simulink model "gm_parallel_prediction_and_cost_function_6phase"  (R2022a)
settings: Solver=FixedStepDiscrete  StartTime=0.0  StopTime=10.0  RelTol=1e-3
undefined symbols (not defined in the file or in its folder): f_c, L_d, L_q, L_x, L_y, p, psi_pm, R_ph
libraries: hdlmdlgenlib x2
(part 5 of 8)

== system gm_parallel_prediction_and_cost_function_6phase/Prediction_and_cost_function/Subsystem/Subsystem3 ==
  SampleTime_div_Ld : Inport  OutDataTypeStr=single  PortDimensions=1  SampleTime=1e-08
  SampleTime_div_Lq : Inport  Port=2  OutDataTypeStr=single  PortDimensions=1  SampleTime=1e-08
  SampleTime_div_Lx : Inport  Port=3  OutDataTypeStr=single  PortDimensions=1  SampleTime=1e-08
  SampleTime_div_Ly : Inport  Port=4  OutDataTypeStr=single  PortDimensions=1  SampleTime=1e-08
  d_phase_voltage_per_switching_state : Inport  Port=5  OutDataTypeStr=single  PortDimensions=1  SampleTime=1e-08
  q_phase_voltage_per_switching_state : Inport  Port=6  OutDataTypeStr=single  PortDimensions=1  SampleTime=1e-08
  x_phase_voltage_per_switching_state : Inport  Port=7  OutDataTypeStr=single  PortDimensions=1  SampleTime=1e-08
  y_phase_voltage_per_switching_state : Inport  Port=8  OutDataTypeStr=single  PortDimensions=1  SampleTime=1e-08
  id_k : Inport  Port=9  OutDataTypeStr=single  PortDimensions=1  SampleTime=1e-08
  iq_k : Inport  Port=10  OutDataTypeStr=single  PortDimensions=1  SampleTime=1e-08
  ix_k : Inport  Port=11  OutDataTypeStr=single  PortDimensions=1  SampleTime=1e-08
  iy_k : Inport  Port=12  OutDataTypeStr=single  PortDimensions=1  SampleTime=1e-08
  psiPM : Inport  Port=13  OutDataTypeStr=single  PortDimensions=1  SampleTime=1e-08
  Lq : Inport  Port=14  OutDataTypeStr=single  PortDimensions=1  SampleTime=1e-08
  Ld : Inport  Port=15  OutDataTypeStr=single  PortDimensions=1  SampleTime=1e-08
  Rs : Inport  Port=16  OutDataTypeStr=single  PortDimensions=1  SampleTime=1e-08
  omega_el : Inport  Port=17  OutDataTypeStr=single  PortDimensions=1  SampleTime=1e-08
  Add : Subsystem
      mask Display: disp('NFP\nadd');
  Add1 : Subsystem
      mask Display: disp('NFP\nadd');
  Add2 : Subsystem
      mask Display: disp('NFP\nadd');
  Add3 : Subsystem
      mask Display: disp('NFP\nadd');
  Add4 : Subsystem
      mask Display: disp('NFP\nadd');
  Product1 : Subsystem
      mask Display: disp('NFP\nmul');
  Product10 : Subsystem
      mask Display: disp('NFP\nmul');
  Product11 : Subsystem
      mask Display: disp('NFP\nmul');
  Product2 : Subsystem
      mask Display: disp('NFP\nmul');
  Product3 : Subsystem
      mask Display: disp('NFP\nmul');
  Product31 : Subsystem
      mask Display: disp('NFP\nmul');
  Product4 : Subsystem
      mask Display: disp('NFP\nmul');
  Product5 : Subsystem
      mask Display: disp('NFP\nmul');
  Product6 : Subsystem
      mask Display: disp('NFP\nmul');
  Product7 : Subsystem
      mask Display: disp('NFP\nmul');
  Product8 : Subsystem
      mask Display: disp('NFP\nmul');
  Product9 : Subsystem
      mask Display: disp('NFP\nmul');
  Subtract1_stage2 : Subsystem
      mask Display: disp('NFP\nadd');
  Subtract1_stage3 : Subsystem
      mask Display: disp('NFP\nadd');
  Subtract2 : Subsystem
      mask Display: disp('NFP\nadd');
  Subtract3 : Subsystem
      mask Display: disp('NFP\nadd');
  Subtract_stage2 : Subsystem
      mask Display: disp('NFP\nadd');
  Subtract_stage3 : Subsystem
      mask Display: disp('NFP\nadd');
  delayMatch : Delay  DelayLength=double(18)  InitialCondition=0  SampleTime=1e-08
  delayMatch1 : Delay  DelayLength=double(18)  InitialCondition=0  SampleTime=1e-08
  delayMatch{2,10..11,13,16..31} (20 alike) : Delay  DelayLength=double(6)  InitialCondition=0  SampleTime=1e-08
  delayMatch{5..9,12,14..15} (8 alike) : Delay  DelayLength=double(12)  InitialCondition=0  SampleTime=1e-08
  delayMatch3 : Delay  DelayLength=double(24)  InitialCondition=0  SampleTime=1e-08
  delayMatch4 : Delay  DelayLength=double(24)  InitialCondition=0  SampleTime=1e-08
  id_13 : Outport  SampleTime=1e-08
  iq_13 : Outport  Port=2  SampleTime=1e-08
  ix_13 : Outport  Port=3  SampleTime=1e-08
  iy_13 : Outport  Port=4  SampleTime=1e-08
  wires:
  delayMatch13/1 -> Subtract_stage3/1(In1)
  delayMatch21/1 -> Subtract1_stage3/1(In1)
  delayMatch14/1 -> Product1/1(In1)
  delayMatch22/1 -> Product4/1(In1)
  delayMatch26/1 -> Product8/1(In1)
  delayMatch30/1 -> Product10/1(In1)
  delayMatch11/1 -> Subtract_stage2/1(In1)
  delayMatch17/1 -> Subtract1_stage2/1(In1)
  delayMatch25/1 -> Subtract2/1(In1)
  delayMatch29/1 -> Subtract3/1(In1)
  delayMatch15/1 -> Add/2(In2)
  delayMatch12/1 -> Product31/2(In2)
  delayMatch27/1 -> Add3/2(In2)
  delayMatch31/1 -> Add4/2(In2)
  delayMatch19/1 -> Add2/1(In1)
  delayMatch20/1 -> Product6/1(In1)
  Add/1(Out1) -> id_13/1
  Add1/1(Out1) -> iq_13/1
  Add2/1(Out1) -> Product6/2(In2)
  Add3/1(Out1) -> ix_13/1
  Add4/1(Out1) -> iy_13/1
  Product1/1(Out1) -> Add/1(In1)
  Product10/1(Out1) -> Add4/1(In1)
  Product11/1(Out1) -> Subtract3/2(In2)
  Product2/1(Out1) -> Subtract_stage2/2(In2)
  Product3/1(Out1) -> Product31/1(In1)
  Product31/1(Out1) -> Subtract_stage3/2(In2)
  Product4/1(Out1) -> Add1/1(In1)
  Product5/1(Out1) -> Subtract1_stage2/2(In2)
  Product6/1(Out1) -> Subtract1_stage3/2(In2)
  Product7/1(Out1) -> Add2/2(In2)
  Product8/1(Out1) -> Add3/1(In1)
  Product9/1(Out1) -> Subtract2/2(In2)
  Subtract_stage2/1(Out1) -> delayMatch13/1
  Subtract_stage3/1(Out1) -> Product1/2(In2)
  Subtract1_stage2/1(Out1) -> delayMatch21/1
  Subtract1_stage3/1(Out1) -> Product4/2(In2)
  Subtract2/1(Out1) -> Product8/2(In2)
  Subtract3/1(Out1) -> Product10/2(In2)
  delayMatch23/1 -> Add1/2(In2)
  delayMatch9/1 -> Product3/2(In2)
  delayMatch18/1 -> Product7/2(In2)
  delayMatch10/1 -> Product2/2(In2)
  delayMatch16/1 -> Product5/2(In2)
  delayMatch/1 -> delayMatch14/1
  delayMatch1/1 -> delayMatch15/1
  delayMatch24/1 -> Product9/2(In2)
  delayMatch2/1 -> delayMatch19/1
  delayMatch3/1 -> delayMatch22/1
  delayMatch4/1 -> delayMatch23/1
  delayMatch28/1 -> Product11/2(In2)
  delayMatch5/1 -> delayMatch26/1
  delayMatch6/1 -> delayMatch27/1
  delayMatch7/1 -> delayMatch30/1
  delayMatch8/1 -> delayMatch31/1
  SampleTime_div_Ld/1 -> delayMatch/1
  SampleTime_div_Lq/1 -> delayMatch3/1
  SampleTime_div_Lx/1 -> delayMatch5/1
  SampleTime_div_Ly/1 -> delayMatch7/1
  d_phase_voltage_per_switching_state/1 -> delayMatch11/1
  q_phase_voltage_per_switching_state/1 -> delayMatch17/1
  x_phase_voltage_per_switching_state/1 -> delayMatch25/1
  y_phase_voltage_per_switching_state/1 -> delayMatch29/1
  id_k/1 -> delayMatch1/1, Product7/1(In1), Product2/1(In1)
  iq_k/1 -> delayMatch4/1, Product5/1(In1), delayMatch12/1
  ix_k/1 -> delayMatch6/1, Product9/1(In1)
  iy_k/1 -> delayMatch8/1, Product11/1(In1)
  psiPM/1 -> delayMatch2/1
  Lq/1 -> delayMatch9/1
  Ld/1 -> delayMatch18/1
  Rs/1 -> delayMatch28/1, delayMatch24/1, delayMatch16/1, delayMatch10/1
  omega_el/1 -> Product3/1(In1), delayMatch20/1

== system gm_parallel_prediction_and_cost_function_6phase/Prediction_and_cost_function/Subsystem/Subsystem4 ==
  SampleTime_div_Ld : Inport  OutDataTypeStr=single  PortDimensions=1  SampleTime=1e-08
  SampleTime_div_Lq : Inport  Port=2  OutDataTypeStr=single  PortDimensions=1  SampleTime=1e-08
  SampleTime_div_Lx : Inport  Port=3  OutDataTypeStr=single  PortDimensions=1  SampleTime=1e-08
  SampleTime_div_Ly : Inport  Port=4  OutDataTypeStr=single  PortDimensions=1  SampleTime=1e-08
  d_phase_voltage_per_switching_state : Inport  Port=5  OutDataTypeStr=single  PortDimensions=1  SampleTime=1e-08
  q_phase_voltage_per_switching_state : Inport  Port=6  OutDataTypeStr=single  PortDimensions=1  SampleTime=1e-08
  x_phase_voltage_per_switching_state : Inport  Port=7  OutDataTypeStr=single  PortDimensions=1  SampleTime=1e-08
  y_phase_voltage_per_switching_state : Inport  Port=8  OutDataTypeStr=single  PortDimensions=1  SampleTime=1e-08
  id_k : Inport  Port=9  OutDataTypeStr=single  PortDimensions=1  SampleTime=1e-08
  iq_k : Inport  Port=10  OutDataTypeStr=single  PortDimensions=1  SampleTime=1e-08
  ix_k : Inport  Port=11  OutDataTypeStr=single  PortDimensions=1  SampleTime=1e-08
  iy_k : Inport  Port=12  OutDataTypeStr=single  PortDimensions=1  SampleTime=1e-08
  psiPM : Inport  Port=13  OutDataTypeStr=single  PortDimensions=1  SampleTime=1e-08
  Lq : Inport  Port=14  OutDataTypeStr=single  PortDimensions=1  SampleTime=1e-08
  Ld : Inport  Port=15  OutDataTypeStr=single  PortDimensions=1  SampleTime=1e-08
  Rs : Inport  Port=16  OutDataTypeStr=single  PortDimensions=1  SampleTime=1e-08
  omega_el : Inport  Port=17  OutDataTypeStr=single  PortDimensions=1  SampleTime=1e-08
  Add : Subsystem
      mask Display: disp('NFP\nadd');
  Add1 : Subsystem
      mask Display: disp('NFP\nadd');
  Add2 : Subsystem
      mask Display: disp('NFP\nadd');
  Add3 : Subsystem
      mask Display: disp('NFP\nadd');
  Add4 : Subsystem
      mask Display: disp('NFP\nadd');
  Product1 : Subsystem
      mask Display: disp('NFP\nmul');
  Product10 : Subsystem
      mask Display: disp('NFP\nmul');
  Product11 : Subsystem
      mask Display: disp('NFP\nmul');
  Product2 : Subsystem
      mask Display: disp('NFP\nmul');
  Product3 : Subsystem
      mask Display: disp('NFP\nmul');
  Product31 : Subsystem
      mask Display: disp('NFP\nmul');
  Product4 : Subsystem
      mask Display: disp('NFP\nmul');
  Product5 : Subsystem
      mask Display: disp('NFP\nmul');
  Product6 : Subsystem
      mask Display: disp('NFP\nmul');
  Product7 : Subsystem
      mask Display: disp('NFP\nmul');
  Product8 : Subsystem
      mask Display: disp('NFP\nmul');
  Product9 : Subsystem
      mask Display: disp('NFP\nmul');
  Subtract1_stage2 : Subsystem
      mask Display: disp('NFP\nadd');
  Subtract1_stage3 : Subsystem
      mask Display: disp('NFP\nadd');
  Subtract2 : Subsystem
      mask Display: disp('NFP\nadd');
  Subtract3 : Subsystem
      mask Display: disp('NFP\nadd');
  Subtract_stage2 : Subsystem
      mask Display: disp('NFP\nadd');
  Subtract_stage3 : Subsystem
      mask Display: disp('NFP\nadd');
  delayMatch : Delay  DelayLength=double(18)  InitialCondition=0  SampleTime=1e-08
  delayMatch1 : Delay  DelayLength=double(18)  InitialCondition=0  SampleTime=1e-08
  delayMatch{2,10..11,13,16..31} (20 alike) : Delay  DelayLength=double(6)  InitialCondition=0  SampleTime=1e-08
  delayMatch{5..9,12,14..15} (8 alike) : Delay  DelayLength=double(12)  InitialCondition=0  SampleTime=1e-08
  delayMatch3 : Delay  DelayLength=double(24)  InitialCondition=0  SampleTime=1e-08
  delayMatch4 : Delay  DelayLength=double(24)  InitialCondition=0  SampleTime=1e-08
  id_12 : Outport  SampleTime=1e-08
  iq_12 : Outport  Port=2  SampleTime=1e-08
  ix_12 : Outport  Port=3  SampleTime=1e-08
  iy_12 : Outport  Port=4  SampleTime=1e-08
  wires:
  delayMatch13/1 -> Subtract_stage3/1(In1)
  delayMatch21/1 -> Subtract1_stage3/1(In1)
  delayMatch14/1 -> Product1/1(In1)
  delayMatch22/1 -> Product4/1(In1)
  delayMatch26/1 -> Product8/1(In1)
  delayMatch30/1 -> Product10/1(In1)
  delayMatch11/1 -> Subtract_stage2/1(In1)
  delayMatch17/1 -> Subtract1_stage2/1(In1)
  delayMatch25/1 -> Subtract2/1(In1)
  delayMatch29/1 -> Subtract3/1(In1)
  delayMatch15/1 -> Add/2(In2)
  delayMatch12/1 -> Product31/2(In2)
  delayMatch27/1 -> Add3/2(In2)
  delayMatch31/1 -> Add4/2(In2)
  delayMatch19/1 -> Add2/1(In1)
  delayMatch20/1 -> Product6/1(In1)
  Add/1(Out1) -> id_12/1
  Add1/1(Out1) -> iq_12/1
  Add2/1(Out1) -> Product6/2(In2)
  Add3/1(Out1) -> ix_12/1
  Add4/1(Out1) -> iy_12/1
  Product1/1(Out1) -> Add/1(In1)
  Product10/1(Out1) -> Add4/1(In1)
  Product11/1(Out1) -> Subtract3/2(In2)
  Product2/1(Out1) -> Subtract_stage2/2(In2)
  Product3/1(Out1) -> Product31/1(In1)
  Product31/1(Out1) -> Subtract_stage3/2(In2)
  Product4/1(Out1) -> Add1/1(In1)
  Product5/1(Out1) -> Subtract1_stage2/2(In2)
  Product6/1(Out1) -> Subtract1_stage3/2(In2)
  Product7/1(Out1) -> Add2/2(In2)
  Product8/1(Out1) -> Add3/1(In1)
  Product9/1(Out1) -> Subtract2/2(In2)
  Subtract_stage2/1(Out1) -> delayMatch13/1
  Subtract_stage3/1(Out1) -> Product1/2(In2)
  Subtract1_stage2/1(Out1) -> delayMatch21/1
  Subtract1_stage3/1(Out1) -> Product4/2(In2)
  Subtract2/1(Out1) -> Product8/2(In2)
  Subtract3/1(Out1) -> Product10/2(In2)
  delayMatch23/1 -> Add1/2(In2)
  delayMatch9/1 -> Product3/2(In2)
  delayMatch18/1 -> Product7/2(In2)
  delayMatch10/1 -> Product2/2(In2)
  delayMatch16/1 -> Product5/2(In2)
  delayMatch/1 -> delayMatch14/1
  delayMatch1/1 -> delayMatch15/1
  delayMatch24/1 -> Product9/2(In2)
  delayMatch2/1 -> delayMatch19/1
  delayMatch3/1 -> delayMatch22/1
  delayMatch4/1 -> delayMatch23/1
  delayMatch28/1 -> Product11/2(In2)
  delayMatch5/1 -> delayMatch26/1
  delayMatch6/1 -> delayMatch27/1
  delayMatch7/1 -> delayMatch30/1
  delayMatch8/1 -> delayMatch31/1
  SampleTime_div_Ld/1 -> delayMatch/1
  SampleTime_div_Lq/1 -> delayMatch3/1
  SampleTime_div_Lx/1 -> delayMatch5/1
  SampleTime_div_Ly/1 -> delayMatch7/1
  d_phase_voltage_per_switching_state/1 -> delayMatch11/1
  q_phase_voltage_per_switching_state/1 -> delayMatch17/1
  x_phase_voltage_per_switching_state/1 -> delayMatch25/1
  y_phase_voltage_per_switching_state/1 -> delayMatch29/1
  id_k/1 -> delayMatch1/1, Product7/1(In1), Product2/1(In1)
  iq_k/1 -> delayMatch4/1, Product5/1(In1), delayMatch12/1
  ix_k/1 -> delayMatch6/1, Product9/1(In1)
  iy_k/1 -> delayMatch8/1, Product11/1(In1)
  psiPM/1 -> delayMatch2/1
  Lq/1 -> delayMatch9/1
  Ld/1 -> delayMatch18/1
  Rs/1 -> delayMatch28/1, delayMatch24/1, delayMatch16/1, delayMatch10/1
  omega_el/1 -> Product3/1(In1), delayMatch20/1

== system gm_parallel_prediction_and_cost_function_6phase/Prediction_and_cost_function/Subsystem/Subsystem5 ==
  SampleTime_div_Ld : Inport  OutDataTypeStr=single  PortDimensions=1  SampleTime=1e-08
  SampleTime_div_Lq : Inport  Port=2  OutDataTypeStr=single  PortDimensions=1  SampleTime=1e-08
  SampleTime_div_Lx : Inport  Port=3  OutDataTypeStr=single  PortDimensions=1  SampleTime=1e-08
  SampleTime_div_Ly : Inport  Port=4  OutDataTypeStr=single  PortDimensions=1  SampleTime=1e-08
  d_phase_voltage_per_switching_state : Inport  Port=5  OutDataTypeStr=single  PortDimensions=1  SampleTime=1e-08
  q_phase_voltage_per_switching_state : Inport  Port=6  OutDataTypeStr=single  PortDimensions=1  SampleTime=1e-08
  x_phase_voltage_per_switching_state : Inport  Port=7  OutDataTypeStr=single  PortDimensions=1  SampleTime=1e-08
  y_phase_voltage_per_switching_state : Inport  Port=8  OutDataTypeStr=single  PortDimensions=1  SampleTime=1e-08
  id_k : Inport  Port=9  OutDataTypeStr=single  PortDimensions=1  SampleTime=1e-08
  iq_k : Inport  Port=10  OutDataTypeStr=single  PortDimensions=1  SampleTime=1e-08
  ix_k : Inport  Port=11  OutDataTypeStr=single  PortDimensions=1  SampleTime=1e-08
  iy_k : Inport  Port=12  OutDataTypeStr=single  PortDimensions=1  SampleTime=1e-08
  psiPM : Inport  Port=13  OutDataTypeStr=single  PortDimensions=1  SampleTime=1e-08
  Lq : Inport  Port=14  OutDataTypeStr=single  PortDimensions=1  SampleTime=1e-08
  Ld : Inport  Port=15  OutDataTypeStr=single  PortDimensions=1  SampleTime=1e-08
  Rs : Inport  Port=16  OutDataTypeStr=single  PortDimensions=1  SampleTime=1e-08
  omega_el : Inport  Port=17  OutDataTypeStr=single  PortDimensions=1  SampleTime=1e-08
  Add : Subsystem
      mask Display: disp('NFP\nadd');
  Add1 : Subsystem
      mask Display: disp('NFP\nadd');
  Add2 : Subsystem
      mask Display: disp('NFP\nadd');
  Add3 : Subsystem
      mask Display: disp('NFP\nadd');
  Add4 : Subsystem
      mask Display: disp('NFP\nadd');
  Product1 : Subsystem
      mask Display: disp('NFP\nmul');
  Product10 : Subsystem
      mask Display: disp('NFP\nmul');
  Product11 : Subsystem
      mask Display: disp('NFP\nmul');
  Product2 : Subsystem
      mask Display: disp('NFP\nmul');
  Product3 : Subsystem
      mask Display: disp('NFP\nmul');
  Product31 : Subsystem
      mask Display: disp('NFP\nmul');
  Product4 : Subsystem
      mask Display: disp('NFP\nmul');
  Product5 : Subsystem
      mask Display: disp('NFP\nmul');
  Product6 : Subsystem
      mask Display: disp('NFP\nmul');
  Product7 : Subsystem
      mask Display: disp('NFP\nmul');
  Product8 : Subsystem
      mask Display: disp('NFP\nmul');
  Product9 : Subsystem
      mask Display: disp('NFP\nmul');
  Subtract1_stage2 : Subsystem
      mask Display: disp('NFP\nadd');
  Subtract1_stage3 : Subsystem
      mask Display: disp('NFP\nadd');
  Subtract2 : Subsystem
      mask Display: disp('NFP\nadd');
  Subtract3 : Subsystem
      mask Display: disp('NFP\nadd');
  Subtract_stage2 : Subsystem
      mask Display: disp('NFP\nadd');
  Subtract_stage3 : Subsystem
      mask Display: disp('NFP\nadd');
  delayMatch : Delay  DelayLength=double(18)  InitialCondition=0  SampleTime=1e-08
  delayMatch1 : Delay  DelayLength=double(18)  InitialCondition=0  SampleTime=1e-08
  delayMatch{2,10..11,13,16..31} (20 alike) : Delay  DelayLength=double(6)  InitialCondition=0  SampleTime=1e-08
  delayMatch{5..9,12,14..15} (8 alike) : Delay  DelayLength=double(12)  InitialCondition=0  SampleTime=1e-08
  delayMatch3 : Delay  DelayLength=double(24)  InitialCondition=0  SampleTime=1e-08
  delayMatch4 : Delay  DelayLength=double(24)  InitialCondition=0  SampleTime=1e-08
  id_11 : Outport  SampleTime=1e-08
  iq_11 : Outport  Port=2  SampleTime=1e-08
  ix_11 : Outport  Port=3  SampleTime=1e-08
  iy_11 : Outport  Port=4  SampleTime=1e-08
  wires:
  delayMatch13/1 -> Subtract_stage3/1(In1)
  delayMatch21/1 -> Subtract1_stage3/1(In1)
  delayMatch14/1 -> Product1/1(In1)
  delayMatch22/1 -> Product4/1(In1)
  delayMatch26/1 -> Product8/1(In1)
  delayMatch30/1 -> Product10/1(In1)
  delayMatch11/1 -> Subtract_stage2/1(In1)
  delayMatch17/1 -> Subtract1_stage2/1(In1)
  delayMatch25/1 -> Subtract2/1(In1)
  delayMatch29/1 -> Subtract3/1(In1)
  delayMatch15/1 -> Add/2(In2)
  delayMatch12/1 -> Product31/2(In2)
  delayMatch27/1 -> Add3/2(In2)
  delayMatch31/1 -> Add4/2(In2)
  delayMatch19/1 -> Add2/1(In1)
  delayMatch20/1 -> Product6/1(In1)
  Add/1(Out1) -> id_11/1
  Add1/1(Out1) -> iq_11/1
  Add2/1(Out1) -> Product6/2(In2)
  Add3/1(Out1) -> ix_11/1
  Add4/1(Out1) -> iy_11/1
  Product1/1(Out1) -> Add/1(In1)
  Product10/1(Out1) -> Add4/1(In1)
  Product11/1(Out1) -> Subtract3/2(In2)
  Product2/1(Out1) -> Subtract_stage2/2(In2)
  Product3/1(Out1) -> Product31/1(In1)
  Product31/1(Out1) -> Subtract_stage3/2(In2)
  Product4/1(Out1) -> Add1/1(In1)
  Product5/1(Out1) -> Subtract1_stage2/2(In2)
  Product6/1(Out1) -> Subtract1_stage3/2(In2)
  Product7/1(Out1) -> Add2/2(In2)
  Product8/1(Out1) -> Add3/1(In1)
  Product9/1(Out1) -> Subtract2/2(In2)
  Subtract_stage2/1(Out1) -> delayMatch13/1
  Subtract_stage3/1(Out1) -> Product1/2(In2)
  Subtract1_stage2/1(Out1) -> delayMatch21/1
  Subtract1_stage3/1(Out1) -> Product4/2(In2)
  Subtract2/1(Out1) -> Product8/2(In2)
  Subtract3/1(Out1) -> Product10/2(In2)
  delayMatch23/1 -> Add1/2(In2)
  delayMatch9/1 -> Product3/2(In2)
  delayMatch18/1 -> Product7/2(In2)
  delayMatch10/1 -> Product2/2(In2)
  delayMatch16/1 -> Product5/2(In2)
  delayMatch/1 -> delayMatch14/1
  delayMatch1/1 -> delayMatch15/1
  delayMatch24/1 -> Product9/2(In2)
  delayMatch2/1 -> delayMatch19/1
  delayMatch3/1 -> delayMatch22/1
  delayMatch4/1 -> delayMatch23/1
  delayMatch28/1 -> Product11/2(In2)
  delayMatch5/1 -> delayMatch26/1
  delayMatch6/1 -> delayMatch27/1
  delayMatch7/1 -> delayMatch30/1
  delayMatch8/1 -> delayMatch31/1
  SampleTime_div_Ld/1 -> delayMatch/1
  SampleTime_div_Lq/1 -> delayMatch3/1
  SampleTime_div_Lx/1 -> delayMatch5/1
  SampleTime_div_Ly/1 -> delayMatch7/1
  d_phase_voltage_per_switching_state/1 -> delayMatch11/1
  q_phase_voltage_per_switching_state/1 -> delayMatch17/1
  x_phase_voltage_per_switching_state/1 -> delayMatch25/1
  y_phase_voltage_per_switching_state/1 -> delayMatch29/1
  id_k/1 -> delayMatch1/1, Product7/1(In1), Product2/1(In1)
  iq_k/1 -> delayMatch4/1, Product5/1(In1), delayMatch12/1
  ix_k/1 -> delayMatch6/1, Product9/1(In1)
  iy_k/1 -> delayMatch8/1, Product11/1(In1)
  psiPM/1 -> delayMatch2/1
  Lq/1 -> delayMatch9/1
  Ld/1 -> delayMatch18/1
  Rs/1 -> delayMatch28/1, delayMatch24/1, delayMatch16/1, delayMatch10/1
  omega_el/1 -> Product3/1(In1), delayMatch20/1

== system gm_parallel_prediction_and_cost_function_6phase/Prediction_and_cost_function/Subsystem/Subsystem6 ==
  SampleTime_div_Ld : Inport  OutDataTypeStr=single  PortDimensions=1  SampleTime=1e-08
  SampleTime_div_Lq : Inport  Port=2  OutDataTypeStr=single  PortDimensions=1  SampleTime=1e-08
  SampleTime_div_Lx : Inport  Port=3  OutDataTypeStr=single  PortDimensions=1  SampleTime=1e-08
  SampleTime_div_Ly : Inport  Port=4  OutDataTypeStr=single  PortDimensions=1  SampleTime=1e-08
  d_phase_voltage_per_switching_state : Inport  Port=5  OutDataTypeStr=single  PortDimensions=1  SampleTime=1e-08
  q_phase_voltage_per_switching_state : Inport  Port=6  OutDataTypeStr=single  PortDimensions=1  SampleTime=1e-08
  x_phase_voltage_per_switching_state : Inport  Port=7  OutDataTypeStr=single  PortDimensions=1  SampleTime=1e-08
  y_phase_voltage_per_switching_state : Inport  Port=8  OutDataTypeStr=single  PortDimensions=1  SampleTime=1e-08
  id_k : Inport  Port=9  OutDataTypeStr=single  PortDimensions=1  SampleTime=1e-08
  iq_k : Inport  Port=10  OutDataTypeStr=single  PortDimensions=1  SampleTime=1e-08
  ix_k : Inport  Port=11  OutDataTypeStr=single  PortDimensions=1  SampleTime=1e-08
  iy_k : Inport  Port=12  OutDataTypeStr=single  PortDimensions=1  SampleTime=1e-08
  psiPM : Inport  Port=13  OutDataTypeStr=single  PortDimensions=1  SampleTime=1e-08
  Lq : Inport  Port=14  OutDataTypeStr=single  PortDimensions=1  SampleTime=1e-08
  Ld : Inport  Port=15  OutDataTypeStr=single  PortDimensions=1  SampleTime=1e-08
  Rs : Inport  Port=16  OutDataTypeStr=single  PortDimensions=1  SampleTime=1e-08
  omega_el : Inport  Port=17  OutDataTypeStr=single  PortDimensions=1  SampleTime=1e-08
  Add : Subsystem
      mask Display: disp('NFP\nadd');
  Add1 : Subsystem
      mask Display: disp('NFP\nadd');
  Add2 : Subsystem
      mask Display: disp('NFP\nadd');
  Add3 : Subsystem
      mask Display: disp('NFP\nadd');
  Add4 : Subsystem
      mask Display: disp('NFP\nadd');
  Product1 : Subsystem
      mask Display: disp('NFP\nmul');
  Product10 : Subsystem
      mask Display: disp('NFP\nmul');
  Product11 : Subsystem
      mask Display: disp('NFP\nmul');
  Product2 : Subsystem
      mask Display: disp('NFP\nmul');
  Product3 : Subsystem
      mask Display: disp('NFP\nmul');
  Product31 : Subsystem
      mask Display: disp('NFP\nmul');
  Product4 : Subsystem
      mask Display: disp('NFP\nmul');
  Product5 : Subsystem
      mask Display: disp('NFP\nmul');
  Product6 : Subsystem
      mask Display: disp('NFP\nmul');
  Product7 : Subsystem
      mask Display: disp('NFP\nmul');
  Product8 : Subsystem
      mask Display: disp('NFP\nmul');
  Product9 : Subsystem
      mask Display: disp('NFP\nmul');
  Subtract1_stage2 : Subsystem
      mask Display: disp('NFP\nadd');
  Subtract1_stage3 : Subsystem
      mask Display: disp('NFP\nadd');
  Subtract2 : Subsystem
      mask Display: disp('NFP\nadd');
  Subtract3 : Subsystem
      mask Display: disp('NFP\nadd');
  Subtract_stage2 : Subsystem
      mask Display: disp('NFP\nadd');
  Subtract_stage3 : Subsystem
      mask Display: disp('NFP\nadd');
  delayMatch : Delay  DelayLength=double(18)  InitialCondition=0  SampleTime=1e-08
  delayMatch1 : Delay  DelayLength=double(18)  InitialCondition=0  SampleTime=1e-08
  delayMatch{2,10..11,13,16..31} (20 alike) : Delay  DelayLength=double(6)  InitialCondition=0  SampleTime=1e-08
  delayMatch{5..9,12,14..15} (8 alike) : Delay  DelayLength=double(12)  InitialCondition=0  SampleTime=1e-08
  delayMatch3 : Delay  DelayLength=double(24)  InitialCondition=0  SampleTime=1e-08
  delayMatch4 : Delay  DelayLength=double(24)  InitialCondition=0  SampleTime=1e-08
  id_10 : Outport  SampleTime=1e-08
  iq_10 : Outport  Port=2  SampleTime=1e-08
  ix_10 : Outport  Port=3  SampleTime=1e-08
  iy_10 : Outport  Port=4  SampleTime=1e-08
  wires:
  delayMatch13/1 -> Subtract_stage3/1(In1)
  delayMatch21/1 -> Subtract1_stage3/1(In1)
  delayMatch14/1 -> Product1/1(In1)
  delayMatch22/1 -> Product4/1(In1)
  delayMatch26/1 -> Product8/1(In1)
  delayMatch30/1 -> Product10/1(In1)
  delayMatch11/1 -> Subtract_stage2/1(In1)
  delayMatch17/1 -> Subtract1_stage2/1(In1)
  delayMatch25/1 -> Subtract2/1(In1)
  delayMatch29/1 -> Subtract3/1(In1)
  delayMatch15/1 -> Add/2(In2)
  delayMatch12/1 -> Product31/2(In2)
  delayMatch27/1 -> Add3/2(In2)
  delayMatch31/1 -> Add4/2(In2)
  delayMatch19/1 -> Add2/1(In1)
  delayMatch20/1 -> Product6/1(In1)
  Add/1(Out1) -> id_10/1
  Add1/1(Out1) -> iq_10/1
  Add2/1(Out1) -> Product6/2(In2)
  Add3/1(Out1) -> ix_10/1
  Add4/1(Out1) -> iy_10/1
  Product1/1(Out1) -> Add/1(In1)
  Product10/1(Out1) -> Add4/1(In1)
  Product11/1(Out1) -> Subtract3/2(In2)
  Product2/1(Out1) -> Subtract_stage2/2(In2)
  Product3/1(Out1) -> Product31/1(In1)
  Product31/1(Out1) -> Subtract_stage3/2(In2)
  Product4/1(Out1) -> Add1/1(In1)
  Product5/1(Out1) -> Subtract1_stage2/2(In2)
  Product6/1(Out1) -> Subtract1_stage3/2(In2)
  Product7/1(Out1) -> Add2/2(In2)
  Product8/1(Out1) -> Add3/1(In1)
  Product9/1(Out1) -> Subtract2/2(In2)
  Subtract_stage2/1(Out1) -> delayMatch13/1
  Subtract_stage3/1(Out1) -> Product1/2(In2)
  Subtract1_stage2/1(Out1) -> delayMatch21/1
  Subtract1_stage3/1(Out1) -> Product4/2(In2)
  Subtract2/1(Out1) -> Product8/2(In2)
  Subtract3/1(Out1) -> Product10/2(In2)
  delayMatch23/1 -> Add1/2(In2)
  delayMatch9/1 -> Product3/2(In2)
  delayMatch18/1 -> Product7/2(In2)
  delayMatch10/1 -> Product2/2(In2)
  delayMatch16/1 -> Product5/2(In2)
  delayMatch/1 -> delayMatch14/1
  delayMatch1/1 -> delayMatch15/1
  delayMatch24/1 -> Product9/2(In2)
  delayMatch2/1 -> delayMatch19/1
  delayMatch3/1 -> delayMatch22/1
  delayMatch4/1 -> delayMatch23/1
  delayMatch28/1 -> Product11/2(In2)
  delayMatch5/1 -> delayMatch26/1
  delayMatch6/1 -> delayMatch27/1
  delayMatch7/1 -> delayMatch30/1
  delayMatch8/1 -> delayMatch31/1
  SampleTime_div_Ld/1 -> delayMatch/1
  SampleTime_div_Lq/1 -> delayMatch3/1
  SampleTime_div_Lx/1 -> delayMatch5/1
  SampleTime_div_Ly/1 -> delayMatch7/1
  d_phase_voltage_per_switching_state/1 -> delayMatch11/1
  q_phase_voltage_per_switching_state/1 -> delayMatch17/1
  x_phase_voltage_per_switching_state/1 -> delayMatch25/1
  y_phase_voltage_per_switching_state/1 -> delayMatch29/1
  id_k/1 -> delayMatch1/1, Product7/1(In1), Product2/1(In1)
  iq_k/1 -> delayMatch4/1, Product5/1(In1), delayMatch12/1
  ix_k/1 -> delayMatch6/1, Product9/1(In1)
  iy_k/1 -> delayMatch8/1, Product11/1(In1)
  psiPM/1 -> delayMatch2/1
  Lq/1 -> delayMatch9/1
  Ld/1 -> delayMatch18/1
  Rs/1 -> delayMatch28/1, delayMatch24/1, delayMatch16/1, delayMatch10/1
  omega_el/1 -> Product3/1(In1), delayMatch20/1

== system gm_parallel_prediction_and_cost_function_6phase/Prediction_and_cost_function/Subsystem/Subsystem7 ==
  SampleTime_div_Ld : Inport  OutDataTypeStr=single  PortDimensions=1  SampleTime=1e-08
  SampleTime_div_Lq : Inport  Port=2  OutDataTypeStr=single  PortDimensions=1  SampleTime=1e-08
  SampleTime_div_Lx : Inport  Port=3  OutDataTypeStr=single  PortDimensions=1  SampleTime=1e-08
  SampleTime_div_Ly : Inport  Port=4  OutDataTypeStr=single  PortDimensions=1  SampleTime=1e-08
  d_phase_voltage_per_switching_state : Inport  Port=5  OutDataTypeStr=single  PortDimensions=1  SampleTime=1e-08
  q_phase_voltage_per_switching_state : Inport  Port=6  OutDataTypeStr=single  PortDimensions=1  SampleTime=1e-08
  x_phase_voltage_per_switching_state : Inport  Port=7  OutDataTypeStr=single  PortDimensions=1  SampleTime=1e-08
  y_phase_voltage_per_switching_state : Inport  Port=8  OutDataTypeStr=single  PortDimensions=1  SampleTime=1e-08
  id_k : Inport  Port=9  OutDataTypeStr=single  PortDimensions=1  SampleTime=1e-08
  iq_k : Inport  Port=10  OutDataTypeStr=single  PortDimensions=1  SampleTime=1e-08
  ix_k : Inport  Port=11  OutDataTypeStr=single  PortDimensions=1  SampleTime=1e-08
  iy_k : Inport  Port=12  OutDataTypeStr=single  PortDimensions=1  SampleTime=1e-08
  psiPM : Inport  Port=13  OutDataTypeStr=single  PortDimensions=1  SampleTime=1e-08
  Lq : Inport  Port=14  OutDataTypeStr=single  PortDimensions=1  SampleTime=1e-08
  Ld : Inport  Port=15  OutDataTypeStr=single  PortDimensions=1  SampleTime=1e-08
  Rs : Inport  Port=16  OutDataTypeStr=single  PortDimensions=1  SampleTime=1e-08
  omega_el : Inport  Port=17  OutDataTypeStr=single  PortDimensions=1  SampleTime=1e-08
  Add : Subsystem
      mask Display: disp('NFP\nadd');
  Add1 : Subsystem
      mask Display: disp('NFP\nadd');
  Add2 : Subsystem
      mask Display: disp('NFP\nadd');
  Add3 : Subsystem
      mask Display: disp('NFP\nadd');
  Add4 : Subsystem
      mask Display: disp('NFP\nadd');
  Product1 : Subsystem
      mask Display: disp('NFP\nmul');
  Product10 : Subsystem
      mask Display: disp('NFP\nmul');
  Product11 : Subsystem
      mask Display: disp('NFP\nmul');
  Product2 : Subsystem
      mask Display: disp('NFP\nmul');
  Product3 : Subsystem
      mask Display: disp('NFP\nmul');
  Product31 : Subsystem
      mask Display: disp('NFP\nmul');
  Product4 : Subsystem
      mask Display: disp('NFP\nmul');
  Product5 : Subsystem
      mask Display: disp('NFP\nmul');
  Product6 : Subsystem
      mask Display: disp('NFP\nmul');
  Product7 : Subsystem
      mask Display: disp('NFP\nmul');
  Product8 : Subsystem
      mask Display: disp('NFP\nmul');
  Product9 : Subsystem
      mask Display: disp('NFP\nmul');
  Subtract1_stage2 : Subsystem
      mask Display: disp('NFP\nadd');
  Subtract1_stage3 : Subsystem
      mask Display: disp('NFP\nadd');
  Subtract2 : Subsystem
      mask Display: disp('NFP\nadd');
  Subtract3 : Subsystem
      mask Display: disp('NFP\nadd');
  Subtract_stage2 : Subsystem
      mask Display: disp('NFP\nadd');
  Subtract_stage3 : Subsystem
      mask Display: disp('NFP\nadd');
  delayMatch : Delay  DelayLength=double(18)  InitialCondition=0  SampleTime=1e-08
  delayMatch1 : Delay  DelayLength=double(18)  InitialCondition=0  SampleTime=1e-08
  delayMatch{2,10..11,13,16..31} (20 alike) : Delay  DelayLength=double(6)  InitialCondition=0  SampleTime=1e-08
  delayMatch{5..9,12,14..15} (8 alike) : Delay  DelayLength=double(12)  InitialCondition=0  SampleTime=1e-08
  delayMatch3 : Delay  DelayLength=double(24)  InitialCondition=0  SampleTime=1e-08
  delayMatch4 : Delay  DelayLength=double(24)  InitialCondition=0  SampleTime=1e-08
  id_9 : Outport  SampleTime=1e-08
  iq_9 : Outport  Port=2  SampleTime=1e-08
  ix_9 : Outport  Port=3  SampleTime=1e-08
  iy_9 : Outport  Port=4  SampleTime=1e-08
  wires:
  delayMatch13/1 -> Subtract_stage3/1(In1)
  delayMatch21/1 -> Subtract1_stage3/1(In1)
  delayMatch14/1 -> Product1/1(In1)
  delayMatch22/1 -> Product4/1(In1)
  delayMatch26/1 -> Product8/1(In1)
  delayMatch30/1 -> Product10/1(In1)
  delayMatch11/1 -> Subtract_stage2/1(In1)
  delayMatch17/1 -> Subtract1_stage2/1(In1)
  delayMatch25/1 -> Subtract2/1(In1)
  delayMatch29/1 -> Subtract3/1(In1)
  delayMatch15/1 -> Add/2(In2)
  delayMatch12/1 -> Product31/2(In2)
  delayMatch27/1 -> Add3/2(In2)
  delayMatch31/1 -> Add4/2(In2)
  delayMatch19/1 -> Add2/1(In1)
  delayMatch20/1 -> Product6/1(In1)
  Add/1(Out1) -> id_9/1
  Add1/1(Out1) -> iq_9/1
  Add2/1(Out1) -> Product6/2(In2)
  Add3/1(Out1) -> ix_9/1
  Add4/1(Out1) -> iy_9/1
  Product1/1(Out1) -> Add/1(In1)
  Product10/1(Out1) -> Add4/1(In1)
  Product11/1(Out1) -> Subtract3/2(In2)
  Product2/1(Out1) -> Subtract_stage2/2(In2)
  Product3/1(Out1) -> Product31/1(In1)
  Product31/1(Out1) -> Subtract_stage3/2(In2)
  Product4/1(Out1) -> Add1/1(In1)
  Product5/1(Out1) -> Subtract1_stage2/2(In2)
  Product6/1(Out1) -> Subtract1_stage3/2(In2)
  Product7/1(Out1) -> Add2/2(In2)
  Product8/1(Out1) -> Add3/1(In1)
  Product9/1(Out1) -> Subtract2/2(In2)
  Subtract_stage2/1(Out1) -> delayMatch13/1
  Subtract_stage3/1(Out1) -> Product1/2(In2)
  Subtract1_stage2/1(Out1) -> delayMatch21/1
  Subtract1_stage3/1(Out1) -> Product4/2(In2)
  Subtract2/1(Out1) -> Product8/2(In2)
  Subtract3/1(Out1) -> Product10/2(In2)
  delayMatch23/1 -> Add1/2(In2)
  delayMatch9/1 -> Product3/2(In2)
  delayMatch18/1 -> Product7/2(In2)
  delayMatch10/1 -> Product2/2(In2)
  delayMatch16/1 -> Product5/2(In2)
  delayMatch/1 -> delayMatch14/1
  delayMatch1/1 -> delayMatch15/1
  delayMatch24/1 -> Product9/2(In2)
  delayMatch2/1 -> delayMatch19/1
  delayMatch3/1 -> delayMatch22/1
  delayMatch4/1 -> delayMatch23/1
  delayMatch28/1 -> Product11/2(In2)
  delayMatch5/1 -> delayMatch26/1
  delayMatch6/1 -> delayMatch27/1
  delayMatch7/1 -> delayMatch30/1
  delayMatch8/1 -> delayMatch31/1
  SampleTime_div_Ld/1 -> delayMatch/1
  SampleTime_div_Lq/1 -> delayMatch3/1
  SampleTime_div_Lx/1 -> delayMatch5/1
  SampleTime_div_Ly/1 -> delayMatch7/1
  d_phase_voltage_per_switching_state/1 -> delayMatch11/1
  q_phase_voltage_per_switching_state/1 -> delayMatch17/1
  x_phase_voltage_per_switching_state/1 -> delayMatch25/1
  y_phase_voltage_per_switching_state/1 -> delayMatch29/1
  id_k/1 -> delayMatch1/1, Product7/1(In1), Product2/1(In1)
  iq_k/1 -> delayMatch4/1, Product5/1(In1), delayMatch12/1
  ix_k/1 -> delayMatch6/1, Product9/1(In1)
  iy_k/1 -> delayMatch8/1, Product11/1(In1)
  psiPM/1 -> delayMatch2/1
  Lq/1 -> delayMatch9/1
  Ld/1 -> delayMatch18/1
  Rs/1 -> delayMatch28/1, delayMatch24/1, delayMatch16/1, delayMatch10/1
  omega_el/1 -> Product3/1(In1), delayMatch20/1

== system gm_parallel_prediction_and_cost_function_6phase/Prediction_and_cost_function/Subsystem/Subsystem8 ==
  SampleTime_div_Ld : Inport  OutDataTypeStr=single  PortDimensions=1  SampleTime=1e-08
  SampleTime_div_Lq : Inport  Port=2  OutDataTypeStr=single  PortDimensions=1  SampleTime=1e-08
  SampleTime_div_Lx : Inport  Port=3  OutDataTypeStr=single  PortDimensions=1  SampleTime=1e-08
  SampleTime_div_Ly : Inport  Port=4  OutDataTypeStr=single  PortDimensions=1  SampleTime=1e-08
  d_phase_voltage_per_switching_state : Inport  Port=5  OutDataTypeStr=single  PortDimensions=1  SampleTime=1e-08
  q_phase_voltage_per_switching_state : Inport  Port=6  OutDataTypeStr=single  PortDimensions=1  SampleTime=1e-08
  x_phase_voltage_per_switching_state : Inport  Port=7  OutDataTypeStr=single  PortDimensions=1  SampleTime=1e-08
  y_phase_voltage_per_switching_state : Inport  Port=8  OutDataTypeStr=single  PortDimensions=1  SampleTime=1e-08
  id_k : Inport  Port=9  OutDataTypeStr=single  PortDimensions=1  SampleTime=1e-08
  iq_k : Inport  Port=10  OutDataTypeStr=single  PortDimensions=1  SampleTime=1e-08
  ix_k : Inport  Port=11  OutDataTypeStr=single  PortDimensions=1  SampleTime=1e-08
  iy_k : Inport  Port=12  OutDataTypeStr=single  PortDimensions=1  SampleTime=1e-08
  psiPM : Inport  Port=13  OutDataTypeStr=single  PortDimensions=1  SampleTime=1e-08
  Lq : Inport  Port=14  OutDataTypeStr=single  PortDimensions=1  SampleTime=1e-08
  Ld : Inport  Port=15  OutDataTypeStr=single  PortDimensions=1  SampleTime=1e-08
  Rs : Inport  Port=16  OutDataTypeStr=single  PortDimensions=1  SampleTime=1e-08
  omega_el : Inport  Port=17  OutDataTypeStr=single  PortDimensions=1  SampleTime=1e-08
  Add : Subsystem
      mask Display: disp('NFP\nadd');
  Add1 : Subsystem
      mask Display: disp('NFP\nadd');
  Add2 : Subsystem
      mask Display: disp('NFP\nadd');
  Add3 : Subsystem
      mask Display: disp('NFP\nadd');
  Add4 : Subsystem
      mask Display: disp('NFP\nadd');
  Product1 : Subsystem
      mask Display: disp('NFP\nmul');
  Product10 : Subsystem
      mask Display: disp('NFP\nmul');
  Product11 : Subsystem
      mask Display: disp('NFP\nmul');
  Product2 : Subsystem
      mask Display: disp('NFP\nmul');
  Product3 : Subsystem
      mask Display: disp('NFP\nmul');
  Product31 : Subsystem
      mask Display: disp('NFP\nmul');
  Product4 : Subsystem
      mask Display: disp('NFP\nmul');
  Product5 : Subsystem
      mask Display: disp('NFP\nmul');
  Product6 : Subsystem
      mask Display: disp('NFP\nmul');
  Product7 : Subsystem
      mask Display: disp('NFP\nmul');
  Product8 : Subsystem
      mask Display: disp('NFP\nmul');
  Product9 : Subsystem
      mask Display: disp('NFP\nmul');
  Subtract1_stage2 : Subsystem
      mask Display: disp('NFP\nadd');
  Subtract1_stage3 : Subsystem
      mask Display: disp('NFP\nadd');
  Subtract2 : Subsystem
      mask Display: disp('NFP\nadd');
  Subtract3 : Subsystem
      mask Display: disp('NFP\nadd');
  Subtract_stage2 : Subsystem
      mask Display: disp('NFP\nadd');
  Subtract_stage3 : Subsystem
      mask Display: disp('NFP\nadd');
  delayMatch : Delay  DelayLength=double(18)  InitialCondition=0  SampleTime=1e-08
  delayMatch1 : Delay  DelayLength=double(18)  InitialCondition=0  SampleTime=1e-08
  delayMatch{2,10..11,13,16..31} (20 alike) : Delay  DelayLength=double(6)  InitialCondition=0  SampleTime=1e-08
  delayMatch{5..9,12,14..15} (8 alike) : Delay  DelayLength=double(12)  InitialCondition=0  SampleTime=1e-08
  delayMatch3 : Delay  DelayLength=double(24)  InitialCondition=0  SampleTime=1e-08
  delayMatch4 : Delay  DelayLength=double(24)  InitialCondition=0  SampleTime=1e-08
  id_8 : Outport  SampleTime=1e-08
  iq_8 : Outport  Port=2  SampleTime=1e-08
  ix_8 : Outport  Port=3  SampleTime=1e-08
  iy_8 : Outport  Port=4  SampleTime=1e-08
  wires:
  delayMatch13/1 -> Subtract_stage3/1(In1)
  delayMatch21/1 -> Subtract1_stage3/1(In1)
  delayMatch14/1 -> Product1/1(In1)
  delayMatch22/1 -> Product4/1(In1)
  delayMatch26/1 -> Product8/1(In1)
  delayMatch30/1 -> Product10/1(In1)
  delayMatch11/1 -> Subtract_stage2/1(In1)
  delayMatch17/1 -> Subtract1_stage2/1(In1)
  delayMatch25/1 -> Subtract2/1(In1)
  delayMatch29/1 -> Subtract3/1(In1)
  delayMatch15/1 -> Add/2(In2)
  delayMatch12/1 -> Product31/2(In2)
  delayMatch27/1 -> Add3/2(In2)
  delayMatch31/1 -> Add4/2(In2)
  delayMatch19/1 -> Add2/1(In1)
  delayMatch20/1 -> Product6/1(In1)
  Add/1(Out1) -> id_8/1
  Add1/1(Out1) -> iq_8/1
  Add2/1(Out1) -> Product6/2(In2)
  Add3/1(Out1) -> ix_8/1
  Add4/1(Out1) -> iy_8/1
  Product1/1(Out1) -> Add/1(In1)
  Product10/1(Out1) -> Add4/1(In1)
  Product11/1(Out1) -> Subtract3/2(In2)
  Product2/1(Out1) -> Subtract_stage2/2(In2)
  Product3/1(Out1) -> Product31/1(In1)
  Product31/1(Out1) -> Subtract_stage3/2(In2)
  Product4/1(Out1) -> Add1/1(In1)
  Product5/1(Out1) -> Subtract1_stage2/2(In2)
  Product6/1(Out1) -> Subtract1_stage3/2(In2)
  Product7/1(Out1) -> Add2/2(In2)
  Product8/1(Out1) -> Add3/1(In1)
  Product9/1(Out1) -> Subtract2/2(In2)
  Subtract_stage2/1(Out1) -> delayMatch13/1
  Subtract_stage3/1(Out1) -> Product1/2(In2)
  Subtract1_stage2/1(Out1) -> delayMatch21/1
  Subtract1_stage3/1(Out1) -> Product4/2(In2)
  Subtract2/1(Out1) -> Product8/2(In2)
  Subtract3/1(Out1) -> Product10/2(In2)
  delayMatch23/1 -> Add1/2(In2)
  delayMatch9/1 -> Product3/2(In2)
  delayMatch18/1 -> Product7/2(In2)
  delayMatch10/1 -> Product2/2(In2)
  delayMatch16/1 -> Product5/2(In2)
  delayMatch/1 -> delayMatch14/1
  delayMatch1/1 -> delayMatch15/1
  delayMatch24/1 -> Product9/2(In2)
  delayMatch2/1 -> delayMatch19/1
  delayMatch3/1 -> delayMatch22/1
  delayMatch4/1 -> delayMatch23/1
  delayMatch28/1 -> Product11/2(In2)
  delayMatch5/1 -> delayMatch26/1
  delayMatch6/1 -> delayMatch27/1
  delayMatch7/1 -> delayMatch30/1
  delayMatch8/1 -> delayMatch31/1
  SampleTime_div_Ld/1 -> delayMatch/1
  SampleTime_div_Lq/1 -> delayMatch3/1
  SampleTime_div_Lx/1 -> delayMatch5/1
  SampleTime_div_Ly/1 -> delayMatch7/1
  d_phase_voltage_per_switching_state/1 -> delayMatch11/1
  q_phase_voltage_per_switching_state/1 -> delayMatch17/1
  x_phase_voltage_per_switching_state/1 -> delayMatch25/1
  y_phase_voltage_per_switching_state/1 -> delayMatch29/1
  id_k/1 -> delayMatch1/1, Product7/1(In1), Product2/1(In1)
  iq_k/1 -> delayMatch4/1, Product5/1(In1), delayMatch12/1
  ix_k/1 -> delayMatch6/1, Product9/1(In1)
  iy_k/1 -> delayMatch8/1, Product11/1(In1)
  psiPM/1 -> delayMatch2/1
  Lq/1 -> delayMatch9/1
  Ld/1 -> delayMatch18/1
  Rs/1 -> delayMatch28/1, delayMatch24/1, delayMatch16/1, delayMatch10/1
  omega_el/1 -> Product3/1(In1), delayMatch20/1

== system gm_parallel_prediction_and_cost_function_6phase/Prediction_and_cost_function/Subsystem/Subsystem9 ==
  SampleTime_div_Ld : Inport  OutDataTypeStr=single  PortDimensions=1  SampleTime=1e-08
  SampleTime_div_Lq : Inport  Port=2  OutDataTypeStr=single  PortDimensions=1  SampleTime=1e-08
  SampleTime_div_Lx : Inport  Port=3  OutDataTypeStr=single  PortDimensions=1  SampleTime=1e-08
  SampleTime_div_Ly : Inport  Port=4  OutDataTypeStr=single  PortDimensions=1  SampleTime=1e-08
  d_phase_voltage_per_switching_state : Inport  Port=5  OutDataTypeStr=single  PortDimensions=1  SampleTime=1e-08
  q_phase_voltage_per_switching_state : Inport  Port=6  OutDataTypeStr=single  PortDimensions=1  SampleTime=1e-08
  x_phase_voltage_per_switching_state : Inport  Port=7  OutDataTypeStr=single  PortDimensions=1  SampleTime=1e-08
  y_phase_voltage_per_switching_state : Inport  Port=8  OutDataTypeStr=single  PortDimensions=1  SampleTime=1e-08
  id_k : Inport  Port=9  OutDataTypeStr=single  PortDimensions=1  SampleTime=1e-08
  iq_k : Inport  Port=10  OutDataTypeStr=single  PortDimensions=1  SampleTime=1e-08
  ix_k : Inport  Port=11  OutDataTypeStr=single  PortDimensions=1  SampleTime=1e-08
  iy_k : Inport  Port=12  OutDataTypeStr=single  PortDimensions=1  SampleTime=1e-08
  psiPM : Inport  Port=13  OutDataTypeStr=single  PortDimensions=1  SampleTime=1e-08
  Lq : Inport  Port=14  OutDataTypeStr=single  PortDimensions=1  SampleTime=1e-08
  Ld : Inport  Port=15  OutDataTypeStr=single  PortDimensions=1  SampleTime=1e-08
  Rs : Inport  Port=16  OutDataTypeStr=single  PortDimensions=1  SampleTime=1e-08
  omega_el : Inport  Port=17  OutDataTypeStr=single  PortDimensions=1  SampleTime=1e-08
  Add : Subsystem
      mask Display: disp('NFP\nadd');
  Add1 : Subsystem
      mask Display: disp('NFP\nadd');
  Add2 : Subsystem
      mask Display: disp('NFP\nadd');
  Add3 : Subsystem
      mask Display: disp('NFP\nadd');
  Add4 : Subsystem
      mask Display: disp('NFP\nadd');
  Product1 : Subsystem
      mask Display: disp('NFP\nmul');
  Product10 : Subsystem
      mask Display: disp('NFP\nmul');
  Product11 : Subsystem
      mask Display: disp('NFP\nmul');
  Product2 : Subsystem
      mask Display: disp('NFP\nmul');
  Product3 : Subsystem
      mask Display: disp('NFP\nmul');
  Product31 : Subsystem
      mask Display: disp('NFP\nmul');
  Product4 : Subsystem
      mask Display: disp('NFP\nmul');
  Product5 : Subsystem
      mask Display: disp('NFP\nmul');
  Product6 : Subsystem
      mask Display: disp('NFP\nmul');
  Product7 : Subsystem
      mask Display: disp('NFP\nmul');
  Product8 : Subsystem
      mask Display: disp('NFP\nmul');
  Product9 : Subsystem
      mask Display: disp('NFP\nmul');
  Subtract1_stage2 : Subsystem
      mask Display: disp('NFP\nadd');
  Subtract1_stage3 : Subsystem
      mask Display: disp('NFP\nadd');
  Subtract2 : Subsystem
      mask Display: disp('NFP\nadd');
  Subtract3 : Subsystem
      mask Display: disp('NFP\nadd');
  Subtract_stage2 : Subsystem
      mask Display: disp('NFP\nadd');
  Subtract_stage3 : Subsystem
      mask Display: disp('NFP\nadd');
  delayMatch : Delay  DelayLength=double(18)  InitialCondition=0  SampleTime=1e-08
  delayMatch1 : Delay  DelayLength=double(18)  InitialCondition=0  SampleTime=1e-08
  delayMatch{2,10..11,13,16..31} (20 alike) : Delay  DelayLength=double(6)  InitialCondition=0  SampleTime=1e-08
  delayMatch{5..9,12,14..15} (8 alike) : Delay  DelayLength=double(12)  InitialCondition=0  SampleTime=1e-08
  delayMatch3 : Delay  DelayLength=double(24)  InitialCondition=0  SampleTime=1e-08
  delayMatch4 : Delay  DelayLength=double(24)  InitialCondition=0  SampleTime=1e-08
  id_7 : Outport  SampleTime=1e-08
  iq_7 : Outport  Port=2  SampleTime=1e-08
  ix_7 : Outport  Port=3  SampleTime=1e-08
  iy_7 : Outport  Port=4  SampleTime=1e-08
  wires:
  delayMatch13/1 -> Subtract_stage3/1(In1)
  delayMatch21/1 -> Subtract1_stage3/1(In1)
  delayMatch14/1 -> Product1/1(In1)
  delayMatch22/1 -> Product4/1(In1)
  delayMatch26/1 -> Product8/1(In1)
  delayMatch30/1 -> Product10/1(In1)
  delayMatch11/1 -> Subtract_stage2/1(In1)
  delayMatch17/1 -> Subtract1_stage2/1(In1)
  delayMatch25/1 -> Subtract2/1(In1)
  delayMatch29/1 -> Subtract3/1(In1)
  delayMatch15/1 -> Add/2(In2)
  delayMatch12/1 -> Product31/2(In2)
  delayMatch27/1 -> Add3/2(In2)
  delayMatch31/1 -> Add4/2(In2)
  delayMatch19/1 -> Add2/1(In1)
  delayMatch20/1 -> Product6/1(In1)
  Add/1(Out1) -> id_7/1
  Add1/1(Out1) -> iq_7/1
  Add2/1(Out1) -> Product6/2(In2)
  Add3/1(Out1) -> ix_7/1
  Add4/1(Out1) -> iy_7/1
  Product1/1(Out1) -> Add/1(In1)
  Product10/1(Out1) -> Add4/1(In1)
  Product11/1(Out1) -> Subtract3/2(In2)
  Product2/1(Out1) -> Subtract_stage2/2(In2)
  Product3/1(Out1) -> Product31/1(In1)
  Product31/1(Out1) -> Subtract_stage3/2(In2)
  Product4/1(Out1) -> Add1/1(In1)
  Product5/1(Out1) -> Subtract1_stage2/2(In2)
  Product6/1(Out1) -> Subtract1_stage3/2(In2)
  Product7/1(Out1) -> Add2/2(In2)
  Product8/1(Out1) -> Add3/1(In1)
  Product9/1(Out1) -> Subtract2/2(In2)
  Subtract_stage2/1(Out1) -> delayMatch13/1
  Subtract_stage3/1(Out1) -> Product1/2(In2)
  Subtract1_stage2/1(Out1) -> delayMatch21/1
  Subtract1_stage3/1(Out1) -> Product4/2(In2)
  Subtract2/1(Out1) -> Product8/2(In2)
  Subtract3/1(Out1) -> Product10/2(In2)
  delayMatch23/1 -> Add1/2(In2)
  delayMatch9/1 -> Product3/2(In2)
  delayMatch18/1 -> Product7/2(In2)
  delayMatch10/1 -> Product2/2(In2)
  delayMatch16/1 -> Product5/2(In2)
  delayMatch/1 -> delayMatch14/1
  delayMatch1/1 -> delayMatch15/1
  delayMatch24/1 -> Product9/2(In2)
  delayMatch2/1 -> delayMatch19/1
  delayMatch3/1 -> delayMatch22/1
  delayMatch4/1 -> delayMatch23/1
  delayMatch28/1 -> Product11/2(In2)
  delayMatch5/1 -> delayMatch26/1
  delayMatch6/1 -> delayMatch27/1
  delayMatch7/1 -> delayMatch30/1
  delayMatch8/1 -> delayMatch31/1
  SampleTime_div_Ld/1 -> delayMatch/1
  SampleTime_div_Lq/1 -> delayMatch3/1
  SampleTime_div_Lx/1 -> delayMatch5/1
  SampleTime_div_Ly/1 -> delayMatch7/1
  d_phase_voltage_per_switching_state/1 -> delayMatch11/1
  q_phase_voltage_per_switching_state/1 -> delayMatch17/1
  x_phase_voltage_per_switching_state/1 -> delayMatch25/1
  y_phase_voltage_per_switching_state/1 -> delayMatch29/1
  id_k/1 -> delayMatch1/1, Product7/1(In1), Product2/1(In1)
  iq_k/1 -> delayMatch4/1, Product5/1(In1), delayMatch12/1
  ix_k/1 -> delayMatch6/1, Product9/1(In1)
  iy_k/1 -> delayMatch8/1, Product11/1(In1)
  psiPM/1 -> delayMatch2/1
  Lq/1 -> delayMatch9/1
  Ld/1 -> delayMatch18/1
  Rs/1 -> delayMatch28/1, delayMatch24/1, delayMatch16/1, delayMatch10/1
  omega_el/1 -> Product3/1(In1), delayMatch20/1

== system gm_parallel_prediction_and_cost_function_6phase/Prediction_and_cost_function/Subsystem/Subsystem/Add ==
  In1 : Inport
  In2 : Inport  Port=2
  Add : Sum  OutDataTypeStr=single  SampleTime=1e-08
  Add_pd1 : Delay  DelayLength=6
  Out1 : Outport
  wires:
  In1/1 -> Add/1
  In2/1 -> Add/2
  Add/1 -> Add_pd1/1
  Add_pd1/1 -> Out1/1

== system gm_parallel_prediction_and_cost_function_6phase/Prediction_and_cost_function/Subsystem/Subsystem/Add1 ==
  In1 : Inport
  In2 : Inport  Port=2
  Add1 : Sum  OutDataTypeStr=single  SampleTime=1e-08
  Add1_pd1 : Delay  DelayLength=6
  Out1 : Outport
  wires:
  In1/1 -> Add1/1
  In2/1 -> Add1/2
  Add1/1 -> Add1_pd1/1
  Add1_pd1/1 -> Out1/1

== system gm_parallel_prediction_and_cost_function_6phase/Prediction_and_cost_function/Subsystem/Subsystem/Add2 ==
  In1 : Inport
  In2 : Inport  Port=2
  Add2 : Sum  OutDataTypeStr=single  SampleTime=1e-08
  Add2_pd1 : Delay  DelayLength=6
  Out1 : Outport
  wires:
  In1/1 -> Add2/1
  In2/1 -> Add2/2
  Add2/1 -> Add2_pd1/1
  Add2_pd1/1 -> Out1/1

== system gm_parallel_prediction_and_cost_function_6phase/Prediction_and_cost_function/Subsystem/Subsystem/Add3 ==
  In1 : Inport
  In2 : Inport  Port=2
  Add3 : Sum  OutDataTypeStr=single  SampleTime=1e-08
  Add3_pd1 : Delay  DelayLength=6
  Out1 : Outport
  wires:
  In1/1 -> Add3/1
  In2/1 -> Add3/2
  Add3/1 -> Add3_pd1/1
  Add3_pd1/1 -> Out1/1

== system gm_parallel_prediction_and_cost_function_6phase/Prediction_and_cost_function/Subsystem/Subsystem/Add4 ==
  In1 : Inport
  In2 : Inport  Port=2
  Add4 : Sum  OutDataTypeStr=single  SampleTime=1e-08
  Add4_pd1 : Delay  DelayLength=6
  Out1 : Outport
  wires:
  In1/1 -> Add4/1
  In2/1 -> Add4/2
  Add4/1 -> Add4_pd1/1
  Add4_pd1/1 -> Out1/1

== system gm_parallel_prediction_and_cost_function_6phase/Prediction_and_cost_function/Subsystem/Subsystem/Product1 ==
  In1 : Inport
  In2 : Inport  Port=2
  Product1 : Product  Inputs=**  OutDataTypeStr=single  SampleTime=1e-08
  Product1_pd1 : Delay  DelayLength=6
  Out1 : Outport
  wires:
  In1/1 -> Product1/1
  In2/1 -> Product1/2
  Product1/1 -> Product1_pd1/1
  Product1_pd1/1 -> Out1/1

== system gm_parallel_prediction_and_cost_function_6phase/Prediction_and_cost_function/Subsystem/Subsystem/Product10 ==
  In1 : Inport
  In2 : Inport  Port=2
  Product10 : Product  Inputs=**  OutDataTypeStr=single  SampleTime=1e-08
  Product10_pd1 : Delay  DelayLength=6
  Out1 : Outport
  wires:
  In1/1 -> Product10/1
  In2/1 -> Product10/2
  Product10/1 -> Product10_pd1/1
  Product10_pd1/1 -> Out1/1

== system gm_parallel_prediction_and_cost_function_6phase/Prediction_and_cost_function/Subsystem/Subsystem/Product11 ==
  In1 : Inport
  In2 : Inport  Port=2
  Product11 : Product  Inputs=**  OutDataTypeStr=single  SampleTime=1e-08
  Product11_pd1 : Delay  DelayLength=6
  Out1 : Outport
  wires:
  In1/1 -> Product11/1
  In2/1 -> Product11/2
  Product11/1 -> Product11_pd1/1
  Product11_pd1/1 -> Out1/1
